simulink model "lift_event"  (R2020b)
settings: Solver=VariableStepAuto  StartTime=0.0  StopTime=10.0  RelTol=1e-3
settings Model: Creator=DELL  LastModifiedBy=DELL

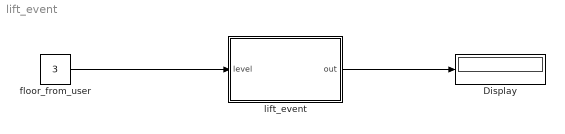
== system lift_event ==
  Display : Display
  floor_from_user : Constant  Value=3
  lift_event : Stateflow chart  TreatAsAtomicUnit=on
  wires:
  floor_from_user/1 -> lift_event/1(level)
  lift_event/1(out) -> Display/1

== stateflow chart lift_event/lift_event ==
  state control [parallel]
    settings: executionOrder=1
    state stop
      out=curr_st;
    state up
      entry:
      curr_st=0;
      du:
      curr_st=curr_st+1;
    state down
      entry:
      curr_st=0;
      du:
      curr_st=curr_st-1;
    (default) -> stop
    stop -> stop [order 3] : [level==curr_st]
    stop -> up [order 2] : [curr_st<level]{send(up,floor_control)}
    stop -> down [order 1] : [curr_st>level]/{send(down,floor_control)}
    up -> stop : [curr_st==level]
    down -> stop : [curr_st==level]
  state floor_control [parallel]
    settings: executionOrder=2
    state floor4
      entry:
      out=4;
    state floor5
      entry:
      out=5;
    state floor2
      entry:
      out=2;
    state floor3
      entry:
      out=3;
    state floor1
      entry:
      curr_st=1;
      out=1;
    (default) -> floor1
    floor5 -> floor5 [order 2] : up
    floor3 -> floor4 [order 1] : up
    floor1 -> floor1 [order 2] : down
    floor4 -> floor5 [order 1] : up
    floor2 -> floor3 [order 1] : up
    floor1 -> floor2 [order 1] : up
    floor3 -> floor2 [order 2] : down
    floor2 -> floor1 [order 2] : down
    floor5 -> floor4 [order 1] : down
    floor4 -> floor3 [order 2] : down
  data: curr_st local =0; level input; out output
  events: up local FUNCTION_CALL_EVENT; down local FUNCTION_CALL_EVENT
